simulink model "sim_onduleurs"  (R2020b)
settings: Solver=ode23tb  StartTime=0.0  StopTime=solver.stop_time  MaxStep=solver.max_step_size  RelTol=solver.tolerance  EnableMultiTasking=on
undefined symbols (not defined in the file or in its folder): E_ch, freq, L_ch, m_hat, modulator_freq, modulator_phase, PWM_gen_carrier_freq, R_ch, saturation_lower, saturation_upper, V_dc, V_dc_sin
libraries: powerlib x13, powerlib_meascontrol x4, simulink x1
settings Model: Creator=ULB  LastModifiedBy=arnaudsaison
settings SolverCC: ZeroCrossControl=EnableAll  ZeroCrossAlgorithm=Adaptive  SolverResetMethod=Robust
settings DataIOCC: LimitDataPoints=on  SaveFormat=Array  SignalLoggingSaveFormat=ModelDataLogs  ReturnWorkspaceOutputs=off
settings OptimizationCC: ExpressionDepthLimit=2147483647  LifeSpan=inf
settings DebuggingCC: UnderspecifiedInitializationDetection=Classic  MergeDetectMultiDrivingBlocksExec=none  SolverPrmCheckMsg=warning  FcnCallInpInsideContextMsg=warning  UnconnectedInputMsg=none  UnconnectedOutputMsg=none  UnconnectedLineMsg=none  StateNameClashWarn=warning  SFUnexpectedBacktrackingDiag=warning  SFNoUnconditionalDefaultTransitionDiag=warning  SFExecutionAtInitializationDiag=none  ArithmeticOperatorsInVariantConditions=warning
settings HardwareCC: ProdBitPerPointer=32  ProdBitPerSizeT=32  ProdBitPerPtrDiffT=32  ProdLargestAtomicFloat=None  ProdIntDivRoundTo=Undefined  ProdEndianess=Unspecified  ProdWordSize=32  ProdHWDeviceType=32-bit Generic
settings ModelReferenceCC: PropagateSignalLabelsOutOfModel=off
settings SFSimCC: SimUseLocalCustomCode=off  CustomCodeUndefinedFunction=UseInterfaceOnly
settings RTWCC: RTWUseLocalCustomCode=off
settings CodeAppCC: StateflowObjectComments=on
settings GRTTargetCC: TargetLangStandard=C89/C90 (ANSI)  CombineOutputUpdateFcns=off  GRTInterface=on
settings ConfigComp: CovMetricSettings=dw  CovSaveCumulativeToWorkspaceVar=on  CovSaveSingleToWorkspaceVar=on  CovExternalEMLEnable=off
settings SimscapeCC: SimscapeNormalizeSystem=off

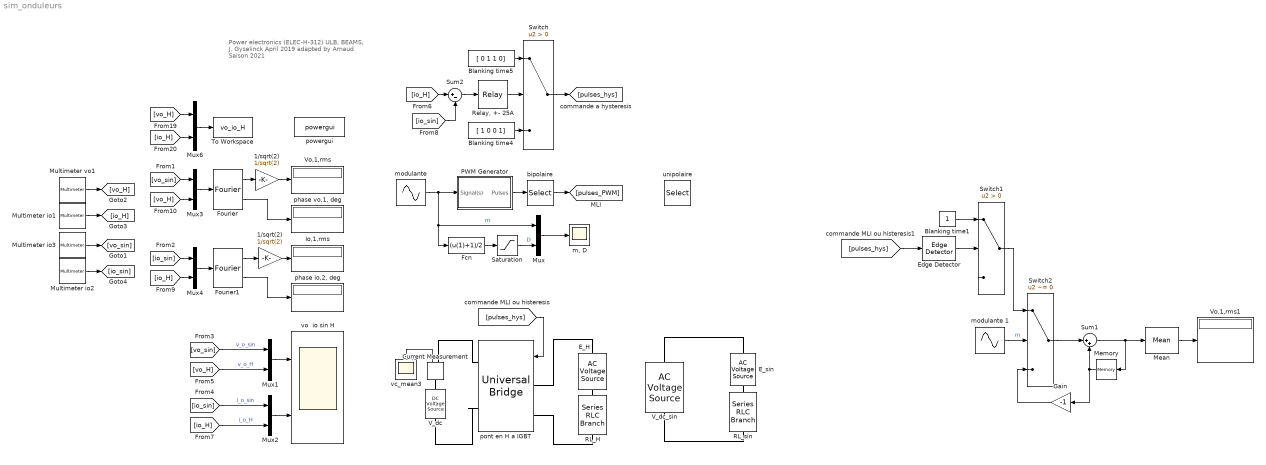
== system sim_onduleurs ==
  note: Power electronics (ELEC-H-312)
      | ULB, BEAMS, J. Gyselinck April 2019
      | adapted by Arnaud Saison 2021
  " RL_sin" : powerlib/Elements/Series RLC Branch  LConnTagsString=__new0  RConnTagsString=__new0  BranchType=RL  Resistance=R_ch  Inductance=L_ch  SetiL0=on  InitialCurrent=0  Capacitance=1e-6  Setx0=off  InitialVoltage=0  Measurements=Branch voltage and current
  1/sqrt(2) : Gain  Gain=1/sqrt(2)
  "1/sqrt(2) " : Gain  Gain=1/sqrt(2)
  Blanking time1 : Constant
  Blanking time4 : Constant  Value=[ 1 0 0 1]
  Blanking time5 : Constant  Value=[ 0 1 1 0]
  Current Measurement : powerlib/Measurements/Current Measurement  PhasorSimulation=off  OutputType=Complex  PSBequivalent=0
  E_H : powerlib/Electrical Sources/AC Voltage Source  Amplitude=E_ch  Phase=0  Frequency=50  SampleTime=0  Measurements=None  BusType=swing  Pref=10e3  Qref=0  Qmin=-inf  Qmax=+inf
  E_sin : powerlib/Electrical Sources/AC Voltage Source  Amplitude=E_ch  Phase=0  Frequency=50  SampleTime=0  Measurements=None  BusType=swing  Pref=10e3  Qref=0  Qmin=-inf  Qmax=+inf
  Edge Detector : powerlib_meascontrol/Logic/Edge Detector  model=Rising  ic=0  Ts=0
      settings: SourceProductBaseCode=PS
  Fcn : Fcn  Expr=(u(1)+1)/2
  Fourier : powerlib_meascontrol/Measurements/Fourier  Freq=freq  n=1  InInit=[0, 0]  Ts=0
  Fourier1 : powerlib_meascontrol/Measurements/Fourier  Freq=freq  n=1  InInit=[0, 0]  Ts=0
  Gain : Gain  Gain=-1
  Io,1,rms : Display
      settings: Format=short_e
  Mean : powerlib_meascontrol/Measurements/Mean  Freq=freq  Vinit=0  Ts=0
  Memory : Memory
  Multimeter io1 : powerlib/Measurements/Multimeter  PhasorSimulation=off  OutputType=Complex  sel=11  L=15  Gain=1  yselected={'Ib: RL_H'};  PSBOutputType=1  PSBequivalent=0  AxesSetting=[0,0.1,-100,100]  Display=0  SavedBlockNames=-11
  Multimeter io2 : powerlib/Measurements/Multimeter  PhasorSimulation=off  OutputType=Complex  sel=10  L=15  Gain=1  yselected="{'Ib:  RL_sin'};"  PSBOutputType=1  PSBequivalent=0  AxesSetting=[0,0.1,-100,100]  Display=0  SavedBlockNames=-11
  Multimeter io3 : powerlib/Measurements/Multimeter  PhasorSimulation=off  OutputType=Complex  sel=9  L=15  Gain=1  yselected={'Usrc: V_dc_sin'};  PSBOutputType=1  PSBequivalent=0  AxesSetting=[0,0.1,-100,100]  Display=0  SavedBlockNames=-11
  Multimeter vo1 : powerlib/Measurements/Multimeter  PhasorSimulation=off  OutputType=Complex  sel=7  L=15  Gain=1  yselected="{'Uab: pont en H  a IGBT'};"  PSBOutputType=1  PSBequivalent=0  AxesSetting=[0,0.1,-100,100]  Display=0  SavedBlockNames=-11
  Mux{,1..4,6} (6 alike) : Mux  Inputs=2
  PWM Generator : Subsystem  AncestorBlock="powerlib_extras/Control  Blocks/PWM Generator"  DialogController=POWERSYS.PowerSysDialog  mask(PWM Generator){GeneratorMode=2-arm  bridge (4 pulses), Fc=PWM_gen_carrier_freq, Internal=off, mIndex=0.4, Freq=60, Phase=0}
      mask prompts: GeneratorMode "Generator Mode"; Fc "Carrier frequency (Hz):"; Internal "Internal generation of modulating signal(s)"; mIndex "Modulation index  (0<m<1) :"; Freq "Frequency of output voltage (Hz)"; Phase "Phase of output voltage (degrees)"
      mask help:
      | This block generates pulses for carrier-based PWM (Pulse Width Modulation), self-commutated IGBTs,GTOs or FETs bridges.
      |
      | Depending on the number of bridge arms selected in the "Generator Mode" parameter, the block can be used either for single-phase or three-phase PWM control.
      mask init:
      | if Freq==0
      |     Phase=90;
      | end
      | switch GeneratorMode
      | case 1,
      |     Internal_Phase=0;
      |    Signal_PortWidth=1;
      |    Select1_Elements=[1 2];
      |    Select1_PortWidth=2;
      |    Select3_Elements=[1 2];
      |    Select3_PortWidth=4;
      | case 2,
      |     Internal_Phase=0;
      |     Signal_PortWidth=1;
      |     Select1_Elements=[1 2];
      |     Select1_PortWidth=2;
      |     Select3_Elements=[1 2 3 4];
      |     Select3_PortWidth=4;
      | case 3,
      |     Internal_Phase=[0 -2*pi/3 2*pi/3];
      |     Signal_PortWidth=3;
      |     Select1_Elements=[1 4 2 5 3 6];
      |     Select1_PortWidth=6;
      |    Select3_Elements=[1 2 3 4 5 6];
      |    Select3_PortWidth=12;
      | case 4,
      |     Internal_Phase=[0 -2*pi/3 2*pi/3];
      |     Signal_PortWidth=3;
      |     Select1_Elements=[1 4 2 5 3 6];
      |     Select1_PortWidth=6;
      |    Select3_Elements=[1 2 3 4 5 6 7 8 9 10 11 12];
      |    Select3_PortWidth=12;
      | end
      | power_initmask();
      mask Help: web(psbhelp)
      mask TypeOptions GeneratorMode: 1-arm  bridge (2 pulses) | 2-arm  bridge (4 pulses) | 3-arm  bridge (6 pulses) | Double 3-arm  bridges (12 pulses)
      mask Callback Internal: p3=get_param(gcb,'Internal');if strcmp(p3,'on');visible={'on','on','on','on','on','on'};else;visible={'on','on','on','off','off','off'};end;set_param(gcb,'MaskVisibilities',visible)
  RL_H : powerlib/Elements/Series RLC Branch  LConnTagsString=__new0  RConnTagsString=__new0  BranchType=RL  Resistance=R_ch  Inductance=L_ch  SetiL0=off  InitialCurrent=0  Capacitance=1e-6  Setx0=off  InitialVoltage=0  Measurements=Branch voltage and current
  "Relay, +- 25A" : Relay  OnSwitchValue=25  OffSwitchValue=-25
  Saturation : Saturate  UpperLimit=saturation_upper  LowerLimit=saturation_lower
  Sum1 : Sum  Inputs=|++
  Sum2 : Sum  Inputs=|+-
  Switch : Switch  Criteria=u2 > Threshold
  Switch1 : Switch  Criteria=u2 > Threshold
  Switch2 : Switch  Criteria=u2 ~= 0
  To Workspace : ToWorkspace  VariableName=vo_io_H  SaveFormat=Structure With Time  SampleTime=-1
      settings: MaxDataPoints=4600*100
  V_dc : powerlib/Electrical Sources/DC Voltage Source  Amplitude=V_dc  Measurements=None
  V_dc_sin : powerlib/Electrical Sources/AC Voltage Source  Amplitude=V_dc_sin * sqrt(2)  Phase=0  Frequency=freq  SampleTime=0  Measurements=Voltage  BusType=swing  Pref=10e3  Qref=0  Qmin=-inf  Qmax=+inf
  Vo,1,rms : Display
      settings: Format=short_e
  Vo,1,rms1 : Display
      settings: Format=short_e
  bipolaire : Selector  InputPortWidth=4  IndexOptions=Index vector (dialog)  Indices=[1 2 2 1]  OutputSizes=1
  "m, D" : Scope
  "modulante " : Sin  Amplitude=m_hat  Frequency=modulator_freq  Phase=modulator_phase  SampleTime=0
  modulante 1 : Sin  Amplitude=m_hat  Frequency=modulator_freq*2  Phase=modulator_phase  SampleTime=0
  "phase io,2, deg" : Display
  "phase vo,1, deg" : Display
  pont en H a IGBT : powerlib/Power Electronics/Universal Bridge  Arms=2  SnubberResistance=1e6  SnubberCapacitance=1e-12  Device=IGBT / Diodes  Ron=1e-3  Lon=0  ForwardVoltages=[ 1 0.8 ]  ForwardVoltage=0  GTOparameters=[ 10e-6 , 20e-6 ]  IGBTparameters=[ 1e-6 , 2e-6 ]  Measurements=All voltages and currents  Measurements_2=None  converterType=Rectifier
  powergui : powerlib/powergui  Priority=1  SimulationMode=Continuous  SampleTime=50e-6  frequency=60  Iterations=50  frequencyindice=50  Pbase=100e6  ErrMax=1e-4  UnitsV=kV  UnitsW=MW  buscounter=0  FunctionMessages=off  echomessages=off  EnableUseOfTLC=off  CurrentSourceSwitches=off  DisableSnubberDevices=on  DisableRonSwitches=on  DisableVfSwitches=on  DisplayEquations=off  AutomaticDiscreteSolvers=off  SolverType=Tustin  Interpol=off  ExternalGateDelay=off  methode=off  Ts=0  x0status=blocks  SPID=on  SwTol=0  HookPort=off  NonlinearTolerance=1e-4  nMaxIteration=100  ContinueOnMaxIteration=off  RestoreLinks=warning  ResistiveCurrentMeasurement=off  Frange=[0:2:500]  Ylog=off  Xlog=on  ShowGrid=off  save=off  variable=ZData  structure=vo_io_H  ZoomFFT=off  StartTime=0.08  cycles=1  DisplayStyle=1  fundamental=50  FreqAxis=on  MaxFrequency=4600  frequencyindicesteady=1  RmsSteady=1  display=off
  unipolaire : Selector  InputPortWidth=4  IndexOptions=Index vector (dialog)  Indices=[1 2 3 4]  OutputSizes=1
  vc_mean3 : Scope
  vo  io sin H : Scope  NumInputPorts=2
  wires:
  Multimeter vo1/1 -> [vo_H]
  Multimeter io1/1 -> [io_H]
  PWM Generator/1(Pulses) -> bipolaire/1
  [io_H] -> Sum2/1
  Sum2/1 -> "Relay, +- 25A"/1
  "Relay, +- 25A"/1 -> Switch/2
  Switch/1 -> [pulses_hys]
  Blanking time5/1 -> Switch/1
  Blanking time4/1 -> Switch/3
  Fcn/1 -> Saturation/1
  Mux/1 -> "m, D"/1
  [vo_sin] -> Mux1/1  "v_o_sin"
  Multimeter io3/1 -> [vo_sin]
  Multimeter io2/1 -> [io_sin]
  [vo_H] -> Mux1/2  "v_o_H"
  [io_sin] -> Mux2/1  "i_o_sin"
  [io_H] -> Mux2/2  "i_o_H"
  [io_sin] -> Sum2/2
  [vo_sin] -> Mux3/1
  [vo_H] -> Mux3/2
  Mux3/1 -> Fourier/1
  [pulses_hys] -> pont en H a IGBT/1
  Current Measurement/1 -> vc_mean3/1
  1/sqrt(2)/1 -> Vo,1,rms/1
  "modulante "/1 -> PWM Generator/1(Signal(s)), Mux/1, Fcn/1  "m"
  Mux6/1 -> To Workspace/1
  [vo_H] -> Mux6/1
  [io_H] -> Mux6/2
  Fourier1/1 -> "1/sqrt(2) "/1
  [io_sin] -> Mux4/1
  [io_H] -> Mux4/2
  Mux4/1 -> Fourier1/1
  "1/sqrt(2) "/1 -> Io,1,rms/1
  Fourier1/2 -> "phase io,2, deg"/1
  bipolaire/1 -> [pulses_PWM]
  Saturation/1 -> Mux/2  "D"
  Fourier/1 -> 1/sqrt(2)/1
  Fourier/2 -> "phase vo,1, deg"/1
  Mux1/1 -> vo  io sin H/1
  Mux2/1 -> vo  io sin H/2
  [pulses_hys] -> Edge Detector/1
  Edge Detector/1 -> Switch1/2
  Mean/1 -> Vo,1,rms1/1
  Memory/1 -> Gain/1, Sum1/2
  Sum1/1 -> Mean/1, Memory/1
  Switch1/1 -> Switch2/1
  modulante 1/1 -> Switch2/2  "m"
  Switch2/1 -> Sum1/1
  Gain/1 -> Switch2/3
  Blanking time1/1 -> Switch1/1
  connections:
  V_dc_sin/LConn1 -- " RL_sin"/RConn1
  E_sin/LConn1 -- " RL_sin"/LConn1
  E_sin/RConn1 -- V_dc_sin/RConn1
  RL_H/RConn1 -- pont en H a IGBT/LConn2
  pont en H a IGBT/RConn2 -- V_dc/LConn1
  RL_H/LConn1 -- E_H/LConn1
  V_dc/RConn1 -- Current Measurement/LConn1
  Current Measurement/RConn1 -- pont en H a IGBT/RConn1
  E_H/RConn1 -- pont en H a IGBT/LConn1

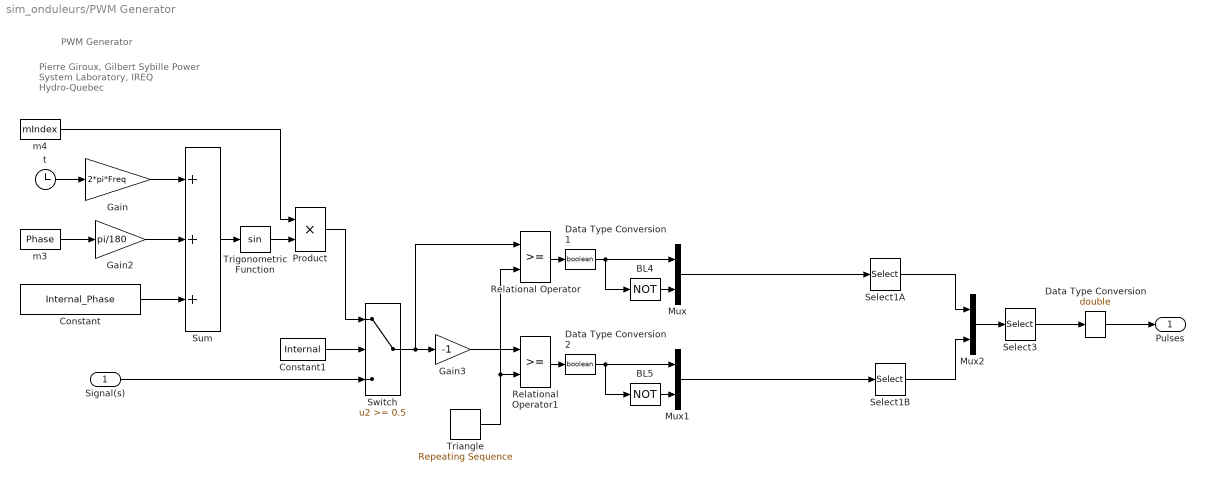
== system sim_onduleurs/PWM Generator ==
  note: PWM Generator
  note: Pierre Giroux, Gilbert Sybille
      | Power System Laboratory, IREQ
      | Hydro-Quebec
  Signal(s) : Inport  PortDimensions=Signal_PortWidth
  BL4 : Logic  Operator=NOT  Inputs=1
  BL5 : Logic  Operator=NOT  Inputs=1
  Constant : Constant  Value=Internal_Phase
  Constant1 : Constant  Value=Internal
  Data Type Conversion : DataTypeConversion  OutDataTypeStr=double  SaturateOnIntegerOverflow=on  RndMeth=Zero
  Data Type Conversion1 : DataTypeConversion  OutDataTypeStr=boolean  SaturateOnIntegerOverflow=on  RndMeth=Zero
  Data Type Conversion2 : DataTypeConversion  OutDataTypeStr=boolean  SaturateOnIntegerOverflow=on  RndMeth=Zero
  Gain : Gain  Gain=2*pi*Freq  SaturateOnIntegerOverflow=on  OutDataTypeStr=Inherit: Same as input  ParamDataTypeStr=Inherit: Same as input
  Gain2 : Gain  Gain=pi/180  SaturateOnIntegerOverflow=on  OutDataTypeStr=Inherit: Same as input  ParamDataTypeStr=Inherit: Same as input
  Gain3 : Gain  Gain=-1  SaturateOnIntegerOverflow=on  OutDataTypeStr=Inherit: Same as input  ParamDataTypeStr=Inherit: Same as input
  Mux : Mux  Inputs=2
  Mux1 : Mux  Inputs=2
  Mux2 : Mux  Inputs=2
  Product : Product  InputSameDT=on  SaturateOnIntegerOverflow=on  OutDataTypeStr=Inherit: Same as first input
  Relational Operator : RelationalOperator  RndMeth=Nearest  InputSameDT=on
  Relational Operator1 : RelationalOperator  RndMeth=Nearest  InputSameDT=on
  Select1A : Selector  InputPortWidth=Select1_PortWidth  IndexOptions=Index vector (dialog)  Indices=Select1_Elements  OutputSizes=1
  Select1B : Selector  InputPortWidth=Select1_PortWidth  IndexOptions=Index vector (dialog)  Indices=Select1_Elements  OutputSizes=1
  Select3 : Selector  InputPortWidth=Select3_PortWidth  IndexOptions=Index vector (dialog)  Indices=Select3_Elements  OutputSizes=1
  Sum : Sum  Inputs=+++  InputSameDT=on  SaturateOnIntegerOverflow=on  OutDataTypeStr=Inherit: Same as first input
  Switch : Switch  Threshold=0.5  InputSameDT=on
  Triangle : simulink/Sources/Repeating Sequence  rep_seq_t=[0 1/Fc/4 3/Fc/4 1/Fc]  rep_seq_y=[0 -1 1 0]
  Trigonometric Function : Trigonometry
  m3 : Constant  Value=Phase
  m4 : Constant  Value=mIndex
  t : Clock
  Pulses : Outport  VectorParamsAs1DForOutWhenUnconnected=off
  wires:
  Data Type Conversion2/1 -> Mux1/1, BL5/1
  Relational Operator1/1 -> Data Type Conversion2/1
  Data Type Conversion1/1 -> Mux/1, BL4/1
  Relational Operator/1 -> Data Type Conversion1/1
  Data Type Conversion/1 -> Pulses/1
  Select3/1 -> Data Type Conversion/1
  t/1 -> Gain/1
  Gain/1 -> Sum/1
  Gain2/1 -> Sum/2
  m3/1 -> Gain2/1
  Constant/1 -> Sum/3
  m4/1 -> Product/1
  Sum/1 -> Trigonometric Function/1
  Trigonometric Function/1 -> Product/2
  Signal(s)/1 -> Switch/3
  Constant1/1 -> Switch/2
  Product/1 -> Switch/1
  Gain3/1 -> Relational Operator1/1
  BL4/1 -> Mux/2
  BL5/1 -> Mux1/2
  Mux/1 -> Select1A/1
  Mux1/1 -> Select1B/1
  Select1A/1 -> Mux2/1
  Select1B/1 -> Mux2/2
  Mux2/1 -> Select3/1
  Switch/1 -> Gain3/1, Relational Operator/1
  Triangle/1 -> Relational Operator1/2, Relational Operator/2
